simulink model "trackloop_tb1"  (R2016a)
settings: Solver=FixedStepDiscrete  SolverMode=SingleTasking  StartTime=0.0  StopTime=5000  RelTol=1e-3
values from neighbouring files (symbols this model uses):
  FINV = true    [trackloop_tb1_main.m]
  x_dir = -1    [trackloop_tb1_main.m]
  x_init = -0.3    [trackloop_tb1_main.m]
  x_step = 0.01    [trackloop_tb1_main.m]
libraries: lib_dsphdlcontrol_v1 x1
settings Model: DataTypeOverride=Off  Creator=mbabst  LastModifiedBy=mbabst
settings DataIOCC: SaveOutput=off  SaveTime=off
settings OptimizationCC: BlockReduction=off  ConditionallyExecuteInputs=off  DefaultParameterBehavior=Inlined
settings DebuggingCC: AlgebraicLoopMsg=error  SingleTaskRateTransMsg=error  StrictBusMsg=ErrorOnBusTreatedAsVector
settings HardwareCC: ProdBitPerPointer=32  ProdLargestAtomicFloat=None  ProdIntDivRoundTo=Undefined  ProdEndianess=Unspecified  ProdWordSize=32  ProdHWDeviceType=ASIC/FPGA->ASIC/FPGA  ProdEqTarget=off
settings GRTTargetCC: GeneratePreprocessorConditionals=Use local settings

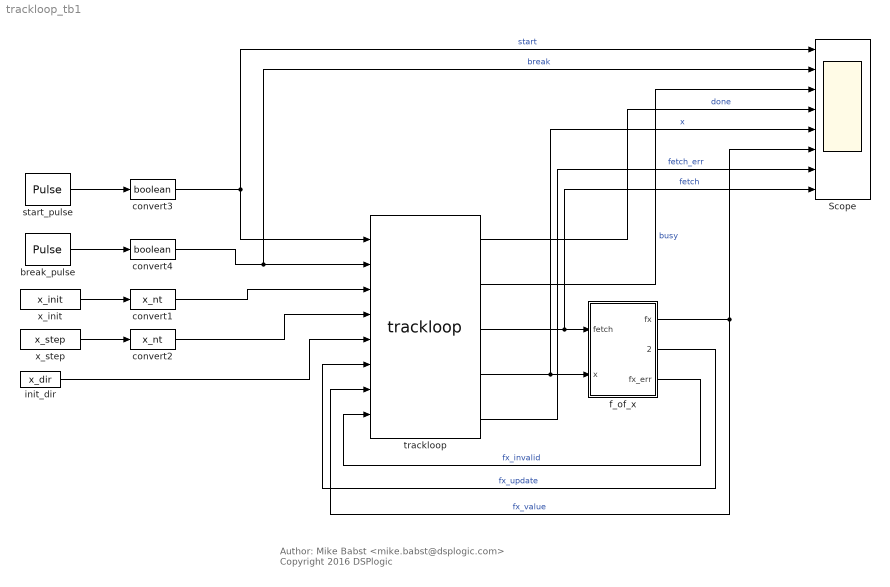
== system trackloop_tb1 ==
  note: Author: Mike Babst <mike.babst@dsplogic.com>
      | Copyright 2016 DSPlogic
  Scope : Scope  NumInputPorts=8
  break_pulse : DiscretePulseGenerator  Period=1e6  PhaseDelay=1000
  convert1 : DataTypeConversion  OutDataTypeStr=x_nt
  convert2 : DataTypeConversion  OutDataTypeStr=x_nt
  convert3 : DataTypeConversion  OutDataTypeStr=boolean
  convert4 : DataTypeConversion  OutDataTypeStr=boolean
  f_of_x : Subsystem
  init_dir : Constant  Value=x_dir  OutDataTypeStr=fixdt(1,2,0)  SampleTime=1
  start_pulse : DiscretePulseGenerator  Period=1e6  PhaseDelay=5
  trackloop : lib_dsphdlcontrol_v1/trackloop  LIMIT=LIMIT  XMIN=XMIN  XMAX=XMAX
  x_init : Constant  Value=x_init  SampleTime=1
  x_step : Constant  Value=x_step  SampleTime=1
  wires:
  start_pulse/1 -> convert3/1
  break_pulse/1 -> convert4/1
  x_init/1 -> convert1/1
  x_step/1 -> convert2/1
  init_dir/1 -> trackloop/5
  convert1/1 -> trackloop/3
  convert2/1 -> trackloop/4
  trackloop/3 -> Scope/8, f_of_x/1(fetch)  "fetch"
  trackloop/4 -> f_of_x/2(x), Scope/5  "x"
  f_of_x/1(fx) -> trackloop/7, Scope/6  "fx_value"
  f_of_x/2(fx_valid) -> trackloop/6  "fx_update"
  f_of_x/3(fx_err) -> trackloop/8  "fx_invalid"
  trackloop/2 -> Scope/3  "busy"
  trackloop/1 -> Scope/4  "done"
  convert3/1 -> trackloop/1, Scope/1  "start"
  convert4/1 -> Scope/2, trackloop/2  "break"
  trackloop/5 -> Scope/7  "fetch_err"

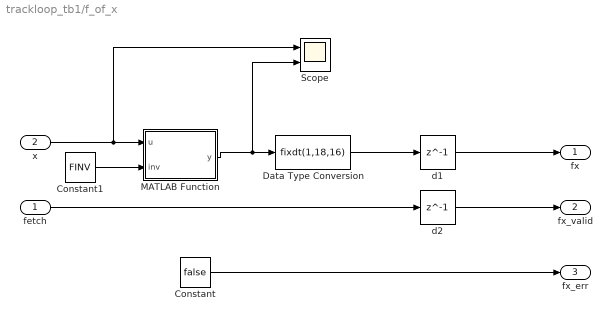
== system trackloop_tb1/f_of_x ==
  fetch : Inport
  x : Inport  Port=2
  Constant : Constant  Value=false  SampleTime=-1
  Constant1 : Constant  Value=FINV  SampleTime=-1
  Data Type Conversion : DataTypeConversion  OutDataTypeStr=fixdt(1,18,16)
  MATLAB Function : MATLAB Function  TreatAsAtomicUnit=on
  Scope : Scope  NumInputPorts=2
  d1 : Delay  DelayLength=1  InitialCondition=0
  d2 : Delay  DelayLength=1  InitialCondition=0
  fx : Outport
  fx_valid : Outport  Port=2
  fx_err : Outport  Port=3
  wires:
  MATLAB Function/1(y) -> Scope/2, Data Type Conversion/1
  x/1 -> MATLAB Function/1(u), Scope/1
  fetch/1 -> d2/1
  d1/1 -> fx/1
  d2/1 -> fx_valid/1
  Constant/1 -> fx_err/1
  Data Type Conversion/1 -> d1/1
  Constant1/1 -> MATLAB Function/2(inv)

== matlab function trackloop_tb1/f_of_x/MATLAB Function ==
  data: u input; y output; inv input
function y = fcn(u, inv)
%#codegen

y = sin(double(u)*2*pi);

if inv
    y = -y;
end
